simulink model "fivelevel_inverter"  (R2020a)
settings: Solver=VariableStepAuto  StartTime=0.0  StopTime=1  RelTol=1e-3
libraries: powerlib x13
settings Model: Creator=hp  LastModifiedBy=hp
settings DebuggingCC: UnconnectedInputMsg=none  UnconnectedOutputMsg=none  UnconnectedLineMsg=none  SFMachineParentedDataDiag=error
settings ModelReferenceCC: EnableRefExpFcnMdlSchedulingChecks=off
settings RTWCC: Description=Generic Real-Time Target

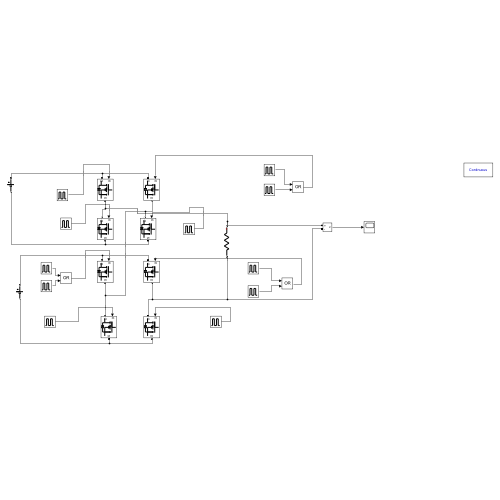
[thumbnail: Simulink's stored preview of the top-level diagram]
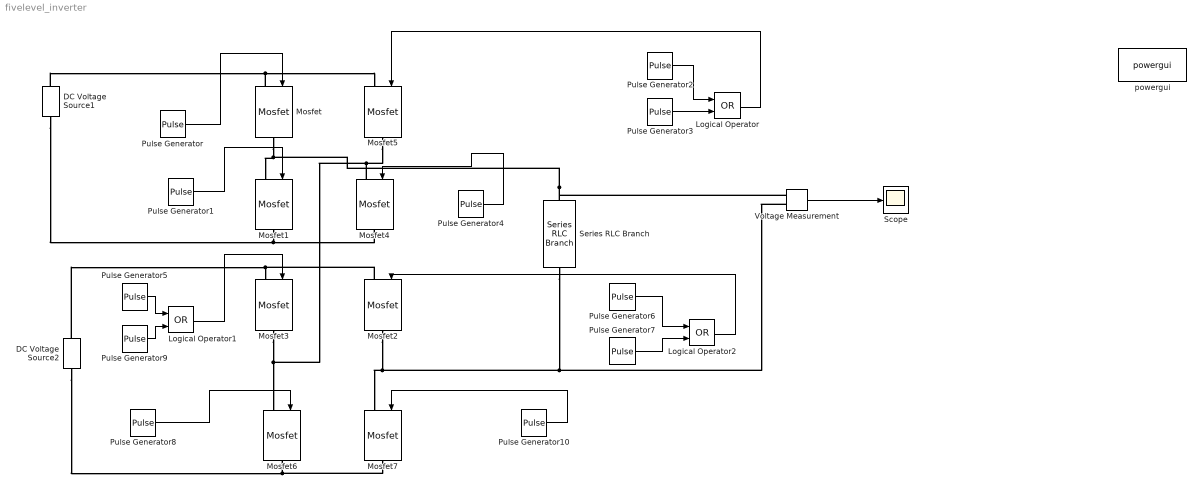
== system fivelevel_inverter ==
  DC Voltage Source1 : powerlib/Electrical Sources/DC Voltage Source  Amplitude=100  Measurements=None
  DC Voltage Source2 : powerlib/Electrical Sources/DC Voltage Source  Amplitude=100  Measurements=None
  Logical Operator : Logic  Operator=OR  AllPortsSameDT=off  OutDataTypeStr=boolean
  Logical Operator1 : Logic  Operator=OR  AllPortsSameDT=off  OutDataTypeStr=boolean
  Logical Operator2 : Logic  Operator=OR  AllPortsSameDT=off  OutDataTypeStr=boolean
  Mosfet{,1..7} (8 alike) : powerlib/Power Electronics/Mosfet  Ron=0.1  Lon=0  Rd=0.01  Vfd=0  IC=0  Rs=1e5  Cs=inf  Measurements=off
  Pulse Generator : DiscretePulseGenerator  PulseType=Time based  Period=0.02  PulseWidth=(5/8)*100  PhaseDelay=(0.02/8)*0
  Pulse Generator1 : DiscretePulseGenerator  PulseType=Time based  Period=0.02  PulseWidth=(3/8)*100  PhaseDelay=(0.02/8)*5
  Pulse Generator10 : DiscretePulseGenerator  PulseType=Time based  Period=0.02  PulseWidth=(1/8)*100  PhaseDelay=(0.02/8)*2
  Pulse Generator2 : DiscretePulseGenerator  PulseType=Time based  Period=0.02  PulseWidth=(1/8)*100  PhaseDelay=(0.02/8)*0
  Pulse Generator3 : DiscretePulseGenerator  PulseType=Time based  Period=0.02  PulseWidth=(4/8)*100  PhaseDelay=(0.02/8)*4
  Pulse Generator4 : DiscretePulseGenerator  PulseType=Time based  Period=0.02  PulseWidth=(3/8)*100  PhaseDelay=(0.02/8)*1
  Pulse Generator5 : DiscretePulseGenerator  PulseType=Time based  Period=0.02  PulseWidth=(6/8)*100  PhaseDelay=(0.02/8)*0
  Pulse Generator6 : DiscretePulseGenerator  PulseType=Time based  Period=0.02  PulseWidth=(2/8)*100  PhaseDelay=(0.02/8)*0
  Pulse Generator7 : DiscretePulseGenerator  PulseType=Time based  Period=0.02  PulseWidth=(5/8)*100  PhaseDelay=(0.02/8)*3
  Pulse Generator8 : DiscretePulseGenerator  PulseType=Time based  Period=0.02  PulseWidth=(1/8)*100  PhaseDelay=(0.02/8)*6
  Pulse Generator9 : DiscretePulseGenerator  PulseType=Time based  Period=0.02  PulseWidth=(1/8)*100  PhaseDelay=(0.02/8)*7
  Scope : Scope
  Series RLC Branch : powerlib/Elements/Series RLC Branch  LConnTagsString=__new0  RConnTagsString=__new0  BranchType=R  Resistance=100  Inductance=1e-3  SetiL0=off  InitialCurrent=0  Capacitance=1e-6  Setx0=off  InitialVoltage=0  Measurements=None
  Voltage Measurement : powerlib/Measurements/Voltage Measurement  PhasorSimulation=off  OutputType=Complex  PSBequivalent=0
  powergui : powerlib/powergui  Priority=1  SimulationMode=Continuous  SampleTime=50e-6  frequency=60  Iterations=50  frequencyindice=0  Pbase=100e6  ErrMax=1e-4  UnitsV=kV  UnitsW=MW  buscounter=0  FunctionMessages=off  echomessages=off  EnableUseOfTLC=off  CurrentSourceSwitches=off  DisableSnubberDevices=off  DisableRonSwitches=off  DisableVfSwitches=off  DisplayEquations=off  AutomaticDiscreteSolvers=off  SolverType=Tustin/Backward Euler (TBE)  Interpol=off  ExternalGateDelay=off  methode=off  Ts=100  x0status=blocks  SPID=on  SwTol=0  HookPort=off  NonlinearTolerance=1e-4  nMaxIteration=100  ContinueOnMaxIteration=off  RestoreLinks=warning  ResistiveCurrentMeasurement=off  Frange=[0:2:500]  Ylog=off  Xlog=on  ShowGrid=off  save=off  variable=ZData  structure=0  ZoomFFT=off  StartTime=0.0  cycles=1  DisplayStyle=1  fundamental=60  FreqAxis=off  MaxFrequency=1000  frequencyindicesteady=1  RmsSteady=1  display=off
  wires:
  Pulse Generator/1 -> Mosfet/1
  Pulse Generator2/1 -> Logical Operator/1
  Pulse Generator3/1 -> Logical Operator/2
  Logical Operator/1 -> Mosfet5/1
  Pulse Generator1/1 -> Mosfet1/1
  Pulse Generator4/1 -> Mosfet4/1
  Pulse Generator5/1 -> Logical Operator1/1
  Pulse Generator9/1 -> Logical Operator1/2
  Logical Operator1/1 -> Mosfet3/1
  Pulse Generator6/1 -> Logical Operator2/1
  Pulse Generator7/1 -> Logical Operator2/2
  Logical Operator2/1 -> Mosfet2/1
  Pulse Generator8/1 -> Mosfet6/1
  Pulse Generator10/1 -> Mosfet7/1
  Voltage Measurement/1 -> Scope/1
  connections:
  Mosfet/RConn1 -- Voltage Measurement/LConn1 -- Series RLC Branch/LConn1 -- Mosfet1/LConn1
  Mosfet1/RConn1 -- Mosfet4/RConn1 -- DC Voltage Source1/LConn1
  Mosfet/LConn1 -- DC Voltage Source1/RConn1 -- Mosfet5/LConn1
  DC Voltage Source2/RConn1 -- Mosfet2/LConn1 -- Mosfet3/LConn1
  DC Voltage Source2/LConn1 -- Mosfet7/RConn1 -- Mosfet6/RConn1
  Mosfet3/RConn1 -- Mosfet4/LConn1 -- Mosfet5/RConn1 -- Mosfet6/LConn1
  Mosfet2/RConn1 -- Voltage Measurement/LConn2 -- Series RLC Branch/RConn1 -- Mosfet7/LConn1
